simulink model "Lab11"  (R2024a)
settings: Solver=VariableStepAuto  StartTime=0.0  StopTime=100  RelTol=1e-3
undefined symbols (not defined in the file or in its folder): C, c1, c2, c3, c4, c5, G, gf, gg, s1, s2, s3, s4, s5, tf0, tg0
libraries: simulink x1
settings Model: Creator=giuse  LastModifiedBy=giuse

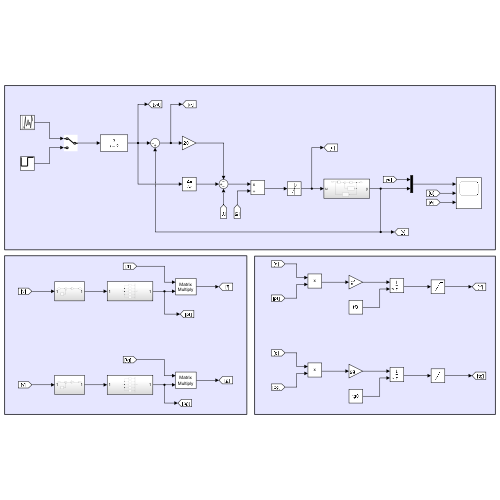
[thumbnail: Simulink's stored preview of the top-level diagram]
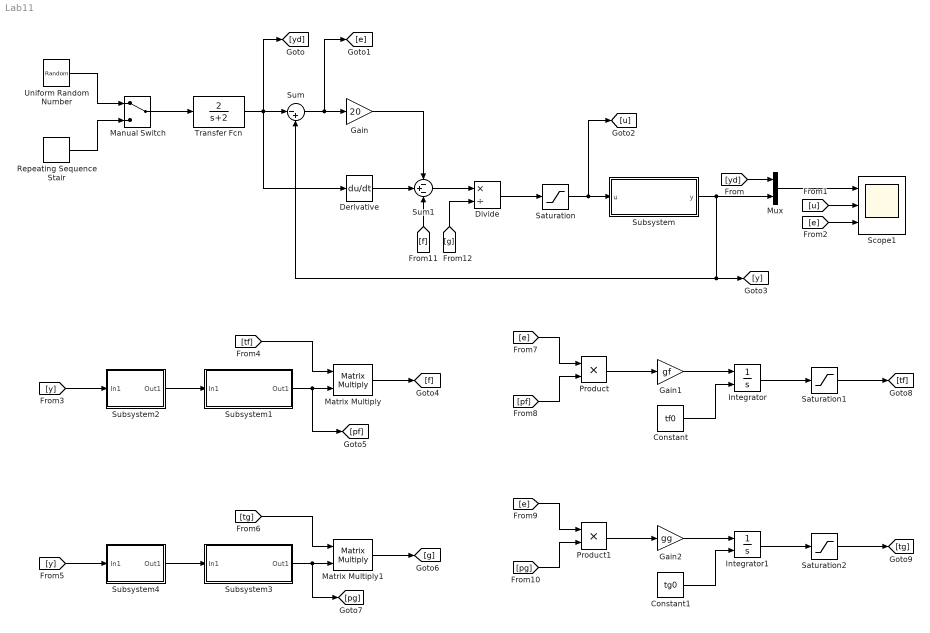
== system Lab11 ==
  Constant : Constant  Value=tf0
  Constant1 : Constant  Value=tg0
  Derivative : Derivative
  Divide : Product  Inputs=*/
  Gain : Gain  Gain=20
  Gain1 : Gain  Gain=gf
  Gain2 : Gain  Gain=gg
  Integrator : Integrator  InitialConditionSource=external
  Integrator1 : Integrator  InitialConditionSource=external
  Manual Switch : ManualSwitch
  Matrix Multiply : Product  Multiplication=Matrix(*)
  Matrix Multiply1 : Product  Multiplication=Matrix(*)
  Mux : Mux  Inputs=2
  Product : Product
  Product1 : Product
  Repeating Sequence Stair : simulink/Sources/Repeating Sequence Stair  OutValues=[20 60].'  tsamp=10  OutMin=[]  OutMax=[]  OutDataTypeStr=double  OutputDataTypeScalingMode=double  OutDataType=fixdt(0,8)  ConRadixGroup=Best Precision: Vector-wise  OutScaling=2^-12
  Saturation : Saturate  UpperLimit=10  LowerLimit=-10
  Saturation1 : Saturate  UpperLimit=30  LowerLimit=-30
  Saturation2 : Saturate  UpperLimit=15  LowerLimit=0.1
  Scope1 : Scope  NumInputPorts=3
  Subsystem : Subsystem
  Subsystem1 : Subsystem
  Subsystem2 : Subsystem
  Subsystem3 : Subsystem
  Subsystem4 : Subsystem
  Sum : Sum  Inputs=|-+
  Sum1 : Sum  Inputs=-+-
  Transfer Fcn : TransferFcn  Numerator=[2]  Denominator=[1 2]
  Uniform Random Number : UniformRandomNumber  Minimum=20  Maximum=60  SampleTime=10
  wires:
  [e] -> Scope1/3
  Subsystem/1(y) -> Sum/2, [y], Mux/2
  Divide/1 -> Saturation/1
  Derivative/1 -> Sum1/2
  Sum1/1 -> Divide/1
  Gain/1 -> Sum1/1
  [u] -> Scope1/2
  Mux/1 -> Scope1/1
  [yd] -> Mux/1
  Saturation/1 -> [u], Subsystem/1(u)
  Uniform Random Number/1 -> Manual Switch/1
  Manual Switch/1 -> Transfer Fcn/1
  Repeating Sequence Stair/1 -> Manual Switch/2
  Transfer Fcn/1 -> [yd], Derivative/1, Sum/1
  Sum/1 -> [e], Gain/1
  Subsystem2/1(Out1) -> Subsystem1/1(In1)
  [y] -> Subsystem2/1(In1)
  Subsystem1/1(Out1) -> [pf], Matrix Multiply/2
  [tf] -> Matrix Multiply/1
  Matrix Multiply/1 -> [f]
  Subsystem3/1(Out1) -> [pg], Matrix Multiply1/2
  [tg] -> Matrix Multiply1/1
  Matrix Multiply1/1 -> [g]
  [y] -> Subsystem4/1(In1)
  Subsystem4/1(Out1) -> Subsystem3/1(In1)
  Product/1 -> Gain1/1
  Gain1/1 -> Integrator/1
  Integrator/1 -> Saturation1/1
  Saturation1/1 -> [tf]
  Constant/1 -> Integrator/2
  [e] -> Product/1
  [pf] -> Product/2
  Gain2/1 -> Integrator1/1
  [e] -> Product1/1
  Product1/1 -> Gain2/1
  [pg] -> Product1/2
  Constant1/1 -> Integrator1/2
  Saturation2/1 -> [tg]
  Integrator1/1 -> Saturation2/1
  [f] -> Sum1/3
  [g] -> Divide/2

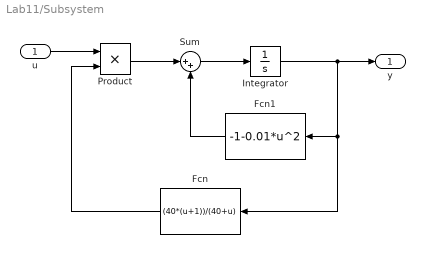
== system Lab11/Subsystem ==
  u : Inport
  Fcn : Fcn  Expr=(40*(u+1))/(40+u)
  Fcn1 : Fcn  Expr=-1-0.01*u^2
  Integrator : Integrator
  Product : Product
  Sum : Sum  Inputs=|++
  y : Outport
  wires:
  u/1 -> Product/1
  Fcn/1 -> Product/2
  Product/1 -> Sum/1
  Fcn1/1 -> Sum/2
  Sum/1 -> Integrator/1
  Integrator/1 -> Fcn/1, Fcn1/1, y/1

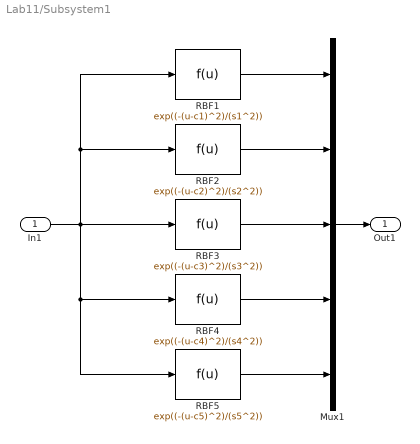
== system Lab11/Subsystem1 ==
  In1 : Inport
  Mux1 : Mux  Inputs=5
  RBF1 : Fcn  Expr=exp((-(u-c1)^2)/(s1^2))
  RBF2 : Fcn  Expr=exp((-(u-c2)^2)/(s2^2))
  RBF3 : Fcn  Expr=exp((-(u-c3)^2)/(s3^2))
  RBF4 : Fcn  Expr=exp((-(u-c4)^2)/(s4^2))
  RBF5 : Fcn  Expr=exp((-(u-c5)^2)/(s5^2))
  Out1 : Outport
  wires:
  RBF1/1 -> Mux1/1
  RBF2/1 -> Mux1/2
  RBF3/1 -> Mux1/3
  RBF4/1 -> Mux1/4
  RBF5/1 -> Mux1/5
  In1/1 -> RBF5/1, RBF4/1, RBF1/1, RBF2/1, RBF3/1
  Mux1/1 -> Out1/1

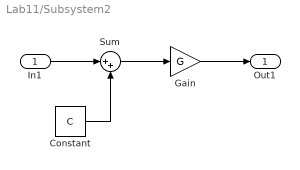
== system Lab11/Subsystem2 ==
  In1 : Inport
  Constant : Constant  Value=C
  Gain : Gain  Gain=G
  Sum : Sum  Inputs=|++
  Out1 : Outport
  wires:
  In1/1 -> Sum/1
  Constant/1 -> Sum/2
  Sum/1 -> Gain/1
  Gain/1 -> Out1/1

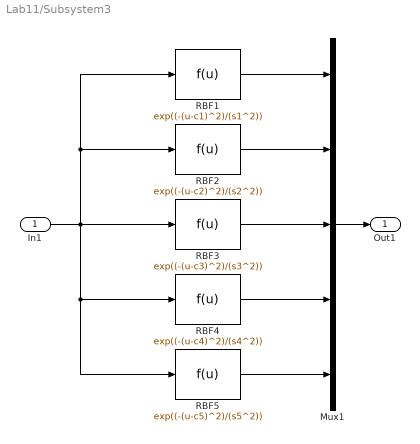
== system Lab11/Subsystem3 ==
  In1 : Inport
  Mux1 : Mux  Inputs=5
  RBF1 : Fcn  Expr=exp((-(u-c1)^2)/(s1^2))
  RBF2 : Fcn  Expr=exp((-(u-c2)^2)/(s2^2))
  RBF3 : Fcn  Expr=exp((-(u-c3)^2)/(s3^2))
  RBF4 : Fcn  Expr=exp((-(u-c4)^2)/(s4^2))
  RBF5 : Fcn  Expr=exp((-(u-c5)^2)/(s5^2))
  Out1 : Outport
  wires:
  RBF1/1 -> Mux1/1
  RBF2/1 -> Mux1/2
  RBF3/1 -> Mux1/3
  RBF4/1 -> Mux1/4
  RBF5/1 -> Mux1/5
  In1/1 -> RBF5/1, RBF4/1, RBF1/1, RBF2/1, RBF3/1
  Mux1/1 -> Out1/1

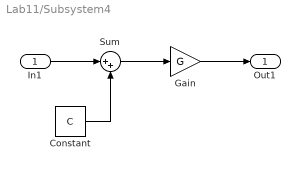
== system Lab11/Subsystem4 ==
  In1 : Inport
  Constant : Constant  Value=C
  Gain : Gain  Gain=G
  Sum : Sum  Inputs=|++
  Out1 : Outport
  wires:
  In1/1 -> Sum/1
  Constant/1 -> Sum/2
  Sum/1 -> Gain/1
  Gain/1 -> Out1/1
